simulink model "PCM_System"  (R2021a)
settings: Solver=VariableStepAuto  StartTime=0.0  StopTime=10.0  RelTol=1e-3
settings Model: Creator=james  LastModifiedBy=james

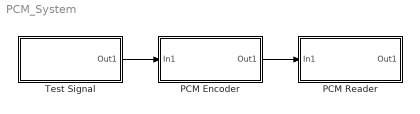
== system PCM_System ==
  PCM Encoder : Subsystem
  PCM Reader : Subsystem
  Test Signal : Subsystem
  wires:
  PCM Encoder/1(Out1) -> PCM Reader/1(In1)
  Test Signal/1(Out1) -> PCM Encoder/1(In1)

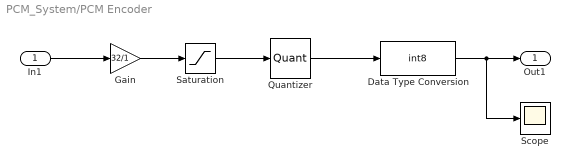
== system PCM_System/PCM Encoder ==
  In1 : Inport
  Data Type Conversion : DataTypeConversion  OutDataTypeStr=int8
  Gain : Gain  Gain=32/1
  Quantizer : Quantizer  QuantizationInterval=1  LinearizeAsGain=off
  Saturation : Saturate  UpperLimit=15  LowerLimit=-15
  Scope : Scope
  Out1 : Outport
  wires:
  In1/1 -> Gain/1
  Data Type Conversion/1 -> Scope/1, Out1/1
  Saturation/1 -> Quantizer/1
  Quantizer/1 -> Data Type Conversion/1
  Gain/1 -> Saturation/1

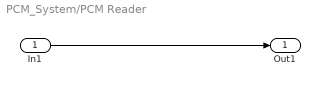
== system PCM_System/PCM Reader ==
  In1 : Inport
  Out1 : Outport
  wires:
  In1/1 -> Out1/1

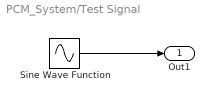
== system PCM_System/Test Signal ==
  Sine Wave Function : Sin  SampleTime=0
  Out1 : Outport
  wires:
  Sine Wave Function/1 -> Out1/1
